simulink model "driver_model_curve"  (R2023b)
settings: Solver=FixedStepAuto  StartTime=0.0  StopTime=50  FixedStep=0.001  MaxStep=0.001  RelTol=1e-3
libraries: Solver_SF x1, slpidlib x1
settings Model: DataTypeOverride=Double  MinMaxOverflowLogging=ForceOff  Creator=황수빈  LastModifiedBy=황수빈

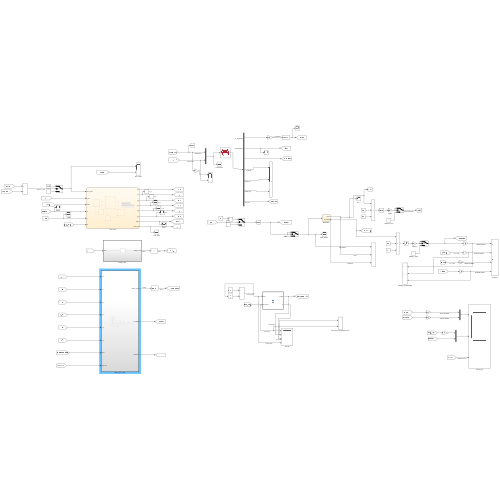
[thumbnail: Simulink's stored preview of the top-level diagram]
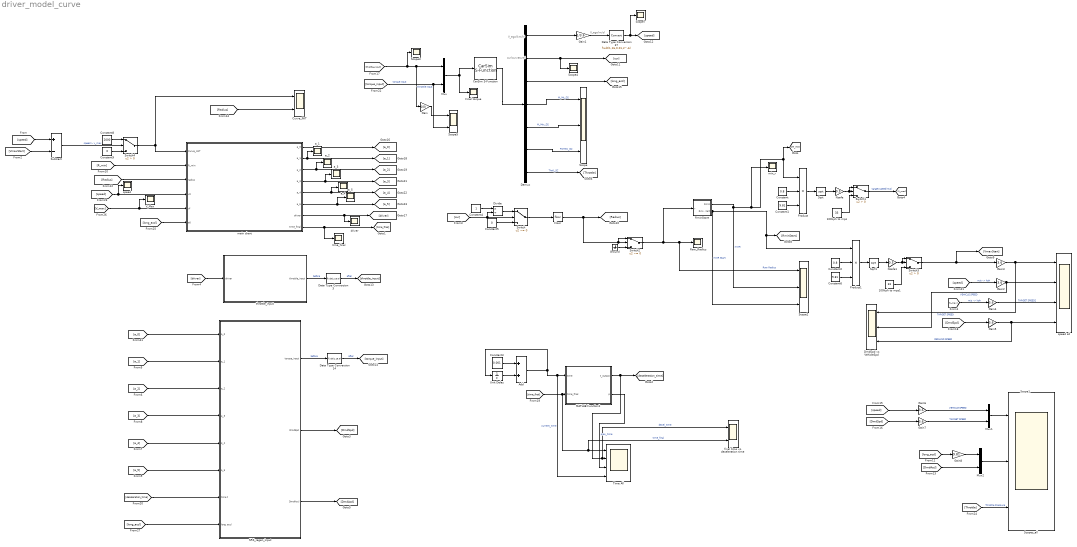
== system driver_model_curve ==
  note: V_ego(km/h)
  note: V_ego(m/s)
  note: cur(curvature)
  100kph to mps : Constant  Value=33
  100kph to mps1 : Constant  Value=33
  Add : Sum
  CarSim S-Function : Solver_SF/CarSim S-Function  Priority=1  SIMFILE=simfile.sim  Run_RTs=off  vs_state_ind=Run  StopMode_ind=Vehicle Model
  Constant : Constant  Value=0.8
  Constant1 : Constant  Value=9.81
  Constant2 : Constant  Value=0.8
  Constant3 : Constant  Value=0.001
  Constant4 : Constant
  Constant5 : Constant  Value=0
  Constant6 : Constant  Value=9.81
  Constant8 : Constant  Value=2000
  Constant9 : Constant  Value=0
  Curve_INIT : Scope  NumInputPorts=2
  Data Type Conversion14 : DataTypeConversion  OutDataTypeStr=fixdt(1,16,0)  RndMeth=Nearest  SaturateOnIntegerOverflow=off
  Data Type Conversion3 : DataTypeConversion  OutDataTypeStr=fixdt(1,16,0)  RndMeth=Nearest  SaturateOnIntegerOverflow=off
  Data Type Conversion37 : DataTypeConversion  OutDataTypeStr=fixdt(1,16,0.01,2^-6)  RndMeth=Simplest  SaturateOnIntegerOverflow=off
  Demux : Demux  Outputs=7
  Divide : Product  Inputs=*/
  DmdSpd vs VehicleSpd : Scope  NumInputPorts=3
  Final torque : Scope
  Floor : Rounding
  Gain : Gain  Gain=100
  Gain1 : Gain  Gain=1/3.6
  Gain{2..7} (6 alike) : Gain  Gain=3.6
  Gain8 : Gain  Gain=9.81
  Ground : Ground
  MATLAB Function1 : MATLAB Function  TreatAsAtomicUnit=on
  Mux : Mux  Inputs=2
  Mux1 : Mux  Inputs=2
  Mux2 : Mux  Inputs=2
  Nsafe : Gain  Gain=0.5
  Nsafe1 : Gain  Gain=0.5
  Product : Product  Inputs=3
  Product1 : Product  Inputs=3
  Raw_Radius : Scope
  RminStore : Stateflow chart  TreatAsAtomicUnit=on
  SRS_regen_input : Subsystem  TreatAsAtomicUnit=on
  Scope : Scope  NumInputPorts=3
  Scope{1,3..4,7} (4 alike) : Scope
  Scope2 : Scope  NumInputPorts=3
  Scope5 : Scope  NumInputPorts=2
  Scopes_all : Scope  NumInputPorts=3
  Sqrt : Sqrt
  Sqrt1 : Sqrt
  Subtract : Sum  Inputs=+-
  Switch : Switch  Criteria=u2 ~= 0  SaturateOnIntegerOverflow=off  InputSameDT=off
  Switch1 : Switch  Criteria=u2 > Threshold  SaturateOnIntegerOverflow=off  InputSameDT=off
  Switch2 : Switch  Criteria=u2 ~= 0  SaturateOnIntegerOverflow=off  InputSameDT=off
  Switch3 : Switch  Criteria=u2 > Threshold  SaturateOnIntegerOverflow=off  InputSameDT=off
  Switch4 : Switch  Criteria=u2 > Threshold  SaturateOnIntegerOverflow=off  InputSameDT=off
  Time All : Scope  NumInputPorts=4
  Unit Delay : UnitDelay  SampleTime=-1  HasFrameUpgradeWarning=on
  V_Max : Scope
  a_{1..5} (5 alike) : Scope
  driver : Scope
  final time vs. deceleration time : Scope  NumInputPorts=2
  main chart : Stateflow chart  TreatAsAtomicUnit=on
  min_r : Scope
  speed : Scope
  speed all : Scope  NumInputPorts=4
  throttle_input : Subsystem  TreatAsAtomicUnit=on  SystemSampleTime=0.01
  time_final : Scope
  wires:
  Switch/1 -> Floor/1
  [cur] -> Switch/2, Divide/2
  Constant5/1 -> Switch/3
  Constant4/1 -> Divide/1
  Divide/1 -> Switch/1
  Gain1/1 -> Data Type Conversion37/1
  Demux/1 -> Gain1/1
  Demux/2 -> Scope4/1, [cur]
  Data Type Conversion37/1 -> Scope7/1, [speed]
  CarSim S-Function/1 -> Demux/1
  [driver] -> throttle_input/1(driver)
  Data Type Conversion3/1 -> [throttle_input]  "after"
  throttle_input/1(throttle_input) -> Data Type Conversion3/1  "before"
  SRS_regen_input/1(torque_input) -> Data Type Conversion14/1  "before"
  [a_2] -> SRS_regen_input/3(a_2)
  Data Type Conversion14/1 -> [torque_input]  "after"
  [a_0] -> SRS_regen_input/1(a_0)
  [a_3] -> SRS_regen_input/4(a_3)
  [a_5] -> SRS_regen_input/6(a_5)
  Demux/3 -> [long_accl]
  [a_1] -> SRS_regen_input/2(a_1)
  [a_4] -> SRS_regen_input/5(a_4)
  Constant8/1 -> Switch4/1
  Constant9/1 -> Switch4/3
  Switch4/1 -> main chart/1(Curve_INIT), Curve_INIT/1
  [speed] -> main chart/4(v0), speed/1
  [V_max] -> V_Max/1, main chart/5(vf)
  main chart/3(a_2) -> a_2/1, [a_2]
  main chart/4(a_3) -> a_3/1, [a_3]
  main chart/5(a_4) -> a_4/1, [a_4]
  main chart/2(a_1) -> a_1/1, [a_1]
  main chart/6(a_5) -> a_5/1, [a_5]
  main chart/7(driver) -> driver/1, [driver]
  [V_max] -> Gain4/1  "m/s -> kph"
  [speed] -> Subtract/1
  [VmaxStart] -> Subtract/2
  Subtract/1 -> Switch4/2  "speed > v_max"
  [R_min] -> main chart/2(R_min)
  main chart/8(time_final) -> time_final/1, [time_final]
  Add/1 -> Unit Delay/1, Time All/4, MATLAB Function1/1(time)  "current_time"
  Gain2/1 -> DmdSpd vs VehicleSpd/2, speed all/2  "VEHICLE SPEED"
  [speed] -> Gain2/1  "m/s -> kph"
  [time_final] -> final time vs. deceleration time/2, Time All/1, MATLAB Function1/2(time_final)  "time_final"
  [Radius] -> main chart/3(radius)
  [torque_input] -> Mux/2, Scope5/2  "torque input"
  [throttle_input] -> Scope3/1, Gain/1, Mux/1  "throttle input"
  Mux/1 -> Final torque/1, CarSim S-Function/1
  Constant3/1 -> Add/1
  Unit Delay/1 -> Add/2
  MATLAB Function1/1(t_output) -> final time vs. deceleration time/1, Time All/2, [deceleration_time]  "decel_time"
  main chart/1(a_0) -> [a_0]
  Constant1/1 -> Product/3
  100kph to mps/1 -> Switch1/3
  Product/1 -> Sqrt/1
  Constant/1 -> Product/2
  Sqrt/1 -> Nsafe/1
  Nsafe/1 -> Switch1/1, Switch1/2
  Switch2/1 -> Scope2/1, Raw_Radius/1, RminStore/1(r)  "Raw Radius"
  Switch1/1 -> [V_max]  "target speed(m/s)"
  Floor/1 -> Switch2/1, Switch2/2, [Radius]
  Ground/1 -> Switch2/3
  MATLAB Function1/2(p) -> Time All/3  "prev_time"
  [deceleration_time] -> SRS_regen_input/7(time t)
  [long_accl] -> main chart/6(a0)
  [long_accl] -> SRS_regen_input/8(long. accl)
  [Radius] -> Curve_INIT/2
  Nsafe1/1 -> Switch3/1, Switch3/2
  100kph to mps1/1 -> Switch3/3
  Constant6/1 -> Product1/3
  Sqrt1/1 -> Nsafe1/1
  Constant2/1 -> Product1/2
  Product1/1 -> Sqrt1/1
  RminStore/1(Rmin) -> min_r/1, Product/1, [R_min], Scope2/2  "minR"
  Switch3/1 -> [VmaxStart], Gain3/1
  Gain3/1 -> DmdSpd vs VehicleSpd/1, speed all/1  "TARGET SPEED"
  SRS_regen_input/2(DmdSpd) -> [DmdSpd]
  [DmdSpd] -> Gain5/1
  Gain5/1 -> DmdSpd vs VehicleSpd/3, speed all/4  "DEMAND SPEED"
  Gain4/1 -> speed all/3  "TARGET SPEED2"
  RminStore/2(RminStart) -> Scope2/3, [RminStart], Product1/1  "minR Start"
  Demux/4 -> Scope/1  "M_Mt_D2"
  Demux/5 -> Scope/2  "M_Mtr_D2"
  Demux/6 -> Scope/3  "PwMtC_D2"
  Demux/7 -> [Throttle]  "Thrtl_SC"
  Gain/1 -> Scope5/1
  SRS_regen_input/3(DmdAccl) -> [DmdAccl]
  [long_accl] -> Gain8/1
  [speed] -> Gain6/1
  [DmdSpd] -> Gain7/1
  Gain7/1 -> Mux1/2  "TARGET SPEED"
  Gain6/1 -> Mux1/1  "VEHICLE SPEED"
  [DmdAccl] -> Mux2/2
  Gain8/1 -> Mux2/1
  Mux1/1 -> Scopes_all/1
  Mux2/1 -> Scopes_all/2
  [Throttle] -> Scopes_all/3  "Throttle Pressure"

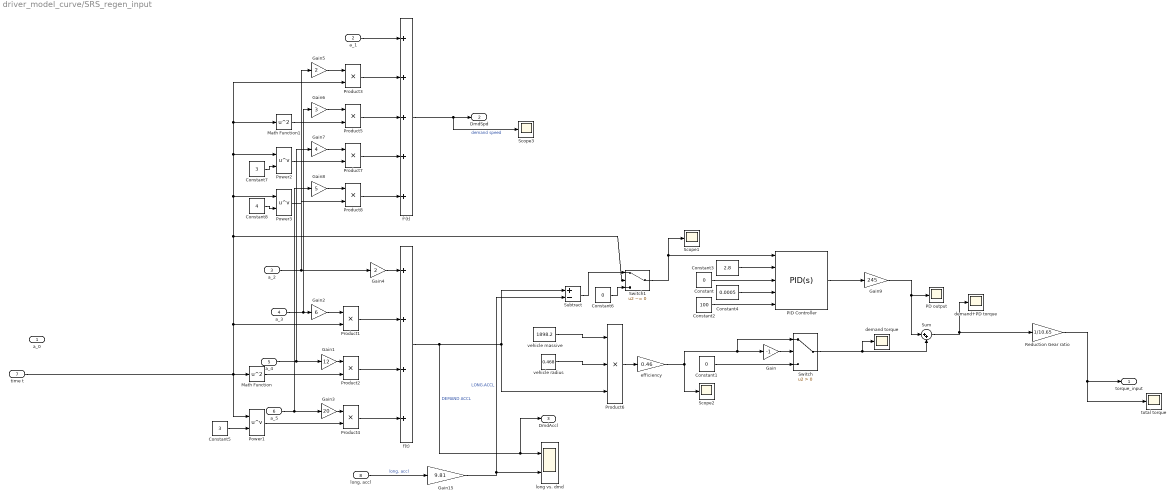
== system driver_model_curve/SRS_regen_input ==
  a_0 : Inport
  a_1 : Inport  Port=2
  a_2 : Inport  Port=3
  a_3 : Inport  Port=4
  a_4 : Inport  Port=5
  a_5 : Inport  Port=6
  time t : Inport  Port=7
  long. accl : Inport  Port=8
  Constant : Constant  Value=0
  Constant1 : Constant  Value=0
  Constant2 : Constant  Value=100
  Constant3 : Constant  Value=2.8
  Constant4 : Constant  Value=0.0005
  Constant5 : Constant  Value=3
  Constant6 : Constant  Value=0
  Constant7 : Constant  Value=3
  Constant8 : Constant  Value=4
  Gain : Gain  Gain=-1
  Gain1 : Gain  Gain=12
  Gain15 : Gain  Gain=9.81
  Gain2 : Gain  Gain=6
  Gain3 : Gain  Gain=20
  Gain4 : Gain  Gain=2
  Gain5 : Gain  Gain=2
  Gain6 : Gain  Gain=3
  Gain7 : Gain  Gain=4
  Gain8 : Gain  Gain=5
  Gain9 : Gain  Gain=245
  Math Function : Math  Operator=square
  Math Function1 : Math  Operator=square
  PD output : Scope
  PID Controller : slpidlib/PID Controller  Controller=PID  Form=Parallel  TimeDomain=Continuous-time  UseExternalTs=off  SampleTime=-1  IntegratorMethod=Forward Euler  FilterMethod=Forward Euler  ControllerParametersSource=external  P=1  I=1  UseKiTs=off  D=0  N=100  UseFilter=on  TunerSelectOption=Transfer Function Based (PID Tuner App)  InitialConditionSource=internal  InitialConditionForIntegrator=0  InitialConditionForFilter=0  DifferentiatorICPrevScaledInput=0  ExternalReset=none  TrackingMode=off  Kt=1  LimitOutput=off  SatLimitsSource=internal  UpperSaturationLimit=inf  LowerSaturationLimit=-inf  LinearizeAsGain=on  AntiWindupMode=none  Kb=1  LimitIntegrator=off  UpperIntegratorSaturationLimit=inf  LowerIntegratorSaturationLimit=-inf  POutMin=[]  POutMax=[]  IOutMin=[]  IOutMax=[]  DOutMin=[]  DOutMax=[]  NOutMin=[]  NOutMax=[]  SumOutMin=[]  SumOutMax=[]  SaturationOutMin=[]  SaturationOutMax=[]  PParamMin=[]  PParamMax=[]  IParamMin=[]  IParamMax=[]  DParamMin=[]  DParamMax=[]  NParamMin=[]  NParamMax=[]  KbParamMin=[]  KbParamMax=[]  KtParamMin=[]  KtParamMax=[]  KbOutMin=[]  KbOutMax=[]  KtOutMin=[]  KtOutMax=[]  IntegratorOutMin=[]  IntegratorOutMax=[]  FilterOutMin=[]  FilterOutMax=[]  SumI1OutMin=[]  SumI1OutMax=[]  SumI2OutMin=[]  SumI2OutMax=[]  SumI3OutMin=[]  SumI3OutMax=[]  SumI4OutMin=[]  SumI4OutMax=[]  SumDOutMin=[]  SumDOutMax=[]  DifferentiatorOutMin=[]  DifferentiatorOutMax=[]  FilterDiffOutCoefMin=[]  FilterDiffOutCoefMax=[]  ReciprocalOutMin=[]  ReciprocalOutMax=[]  SumDenOutMin=[]  SumDenOutMax=[]  SumNumOutMin=[]  SumNumOutMax=[]  DivideOutMin=[]  DivideOutMax=[]  UdiffTsProdOutMin=[]  UdiffTsProdOutMax=[]  NTsProdOutMin=[]  NTsProdOutMax=[]  UintegralTsProdOutMin=[]  UintegralTsProdOutMax=[]  UngainTsProdOutMin=[]  UngainTsProdOutMax=[]  ClampingZeroOutDataTypeStr=Inherit: Inherit via back propagation  ClampingZeroOutMin=[]  ClampingZeroOutMax=[]  FilterDenConstantOutDataTypeStr=Inherit: Inherit via back propagation  FilterDenConstantOutMin=[]  FilterDenConstantOutMax=[]  PCopyOutDataTypeStr=Inherit: Inherit via back propagation  PCopyOutMin=[]  PCopyOutMax=[]  NCopyOutDataTypeStr=Inherit: Inherit via back propagation  NCopyOutMin=[]  NCopyOutMax=[]  IntegratorContinuousStateAttributes=''  IntegratorStateMustResolveToSignalObject=off  IntegratorRTWStateStorageClass=Auto  FilterContinuousStateAttributes=''  FilterStateMustResolveToSignalObject=off  FilterRTWStateStorageClass=Auto  ParallelPVariant=ExternalParameters  IdealPVariant=Disabled  IVariant=ExternalParameters  DVariant=ExternalParameters  IntegratorVariant=Continuous  SatVariant=Disabled  AWVariant=Passthrough  PCopyVariant=Disabled  TRVariant=Disabled  FdbkBlocksVariant=Forward  IdealPFdbkVariant=Disabled  SatFdbkVariant=Disabled  DerivativeFilterVariant=ContFilter  NVariant=ExternalParameters  NCopyVariant=Disabled  FilterICVariant=InternalICsFilter  IntegratorICVariant=InternalICs  ExternalResetVariant=Disabled  TRSumVariant=Passthrough  SumFdbkVariant=Disabled  SumVariant=Sum_PID  TsampFilterVariant=InternalTs  TsampNgainVariant=Passthrough  TsampIntegralVariant=Disabled_SignalSpec  ExternalSaturationOutDataTypeStr=Inherit: Same as second input
  Power1 : Math  Operator=pow
  Power2 : Math  Operator=pow
  Power3 : Math  Operator=pow
  Product{1..5,7..8} (7 alike) : Product
  Product6 : Product  Inputs=3
  Reduction Gear ratio : Gain  Gain=1/10.65
  Scope1 : Scope
  Scope2 : Scope
  Scope3 : Scope
  Subtract : Sum  Inputs=+-
  Sum : Sum  Inputs=|++
  Switch : Switch  Criteria=u2 > Threshold  SaturateOnIntegerOverflow=off  InputSameDT=off
  Switch1 : Switch  Criteria=u2 ~= 0  SaturateOnIntegerOverflow=off  InputSameDT=off
  demand torque : Scope
  demand+PD torque : Scope
  efficiency : Gain  Gain=0.46
  f'(t) : Sum  Inputs=5
  f(t) : Sum  Inputs=4
  long vs. dmd : Scope  NumInputPorts=2
  total torque : Scope
  vehicle massive : Constant  Value=1898.2
  vehicle radius : Constant  Value=0.468
  torque_input : Outport
  DmdSpd : Outport  Port=2
  DmdAccl : Outport  Port=3
  wires:
  time t/1 -> Power3/1, Power2/1, Math Function1/1, Product3/2, Switch1/2, Product1/2, Power1/1, Math Function/1
  Constant5/1 -> Power1/2
  Product2/1 -> f(t)/3
  Product4/1 -> f(t)/4
  Power1/1 -> Product4/2
  Math Function/1 -> Product2/2
  Product6/1 -> efficiency/1
  efficiency/1 -> Scope2/1, Switch/1, Gain/1
  Constant1/1 -> Switch/3
  Gain/1 -> Switch/2
  f(t)/1 -> Product6/3, Subtract/1, DmdAccl/1, long vs. dmd/1  "DEMAND ACCL"
  a_2/1 -> Gain4/1, Gain5/1
  a_4/1 -> Gain1/1, Gain7/1
  Gain1/1 -> Product2/1
  a_5/1 -> Gain8/1, Gain3/1
  Gain3/1 -> Product4/1
  Gain4/1 -> f(t)/1
  a_3/1 -> Gain6/1, Gain2/1
  Gain2/1 -> Product1/1
  Product1/1 -> f(t)/2
  long. accl/1 -> Gain15/1  "long. accl"
  Subtract/1 -> Switch1/1
  Switch1/1 -> PID Controller/1, Scope1/1
  Constant6/1 -> Switch1/3
  Constant2/1 -> PID Controller/5
  Constant4/1 -> PID Controller/4
  Constant/1 -> PID Controller/3
  Constant3/1 -> PID Controller/2
  PID Controller/1 -> Gain9/1
  a_1/1 -> f'(t)/1
  Product3/1 -> f'(t)/2
  Product5/1 -> f'(t)/3
  Product7/1 -> f'(t)/4
  Product8/1 -> f'(t)/5
  Gain5/1 -> Product3/1
  Gain6/1 -> Product5/1
  Gain7/1 -> Product7/1
  Gain8/1 -> Product8/1
  f'(t)/1 -> Scope3/1, DmdSpd/1  "demand speed"
  Math Function1/1 -> Product5/2
  Power2/1 -> Product7/2
  Power3/1 -> Product8/2
  Constant7/1 -> Power2/2
  Constant8/1 -> Power3/2
  Switch/1 -> Sum/2, demand torque/1
  Gain15/1 -> Subtract/2, long vs. dmd/2  "LONG.ACCL"
  vehicle radius/1 -> Product6/2
  vehicle massive/1 -> Product6/1
  Sum/1 -> Reduction Gear ratio/1, demand+PD torque/1
  Gain9/1 -> PD output/1, Sum/1
  Reduction Gear ratio/1 -> total torque/1, torque_input/1

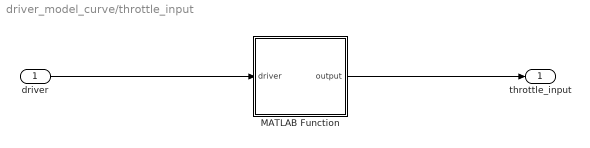
== system driver_model_curve/throttle_input ==
  driver : Inport
  MATLAB Function : MATLAB Function  TreatAsAtomicUnit=on
  throttle_input : Outport
  wires:
  driver/1 -> MATLAB Function/1(driver)
  MATLAB Function/1(output) -> throttle_input/1

== matlab function driver_model_curve/MATLAB Function1 ==
  data: time input; t_output output; time_final input; p output
function [t_output, p] = fcn(time, time_final)
    persistent prev_time;  % 이전 시간 저장용 변수
    if isempty(prev_time)
        prev_time = time;  % 초기화, 첫 호출 시 현재 시간으로 설정
    end

    % time이 time_final에 도달하면 prev_time을 초기화
    if (time - prev_time) < time_final 
        t_output = (time - prev_time);  % time_final에 도달하기 전까지의 값
        p = prev_time;

    
    elseif (time - prev_time) == time_final 
        t_output = 0;  % time_final에 도달하기 전까지의 값
        p = prev_time;

    else
        prev_time = time;  % 새로운 loop 시작 (time_final 도달 후 초기화)
        t_output = 0;  % time_final 도달 후 초기화된 slow_time
        p = prev_time;

    end

end

== matlab function driver_model_curve/throttle_input/MATLAB Function ==
  data: driver input; output output
function output = driver_function(driver)
    switch driver
        case 0
            output = 0;
        case 1
            output = 0.4;
        case 2
            output = 0.04;
        otherwise
            output = 0.4;
    end
end

== stateflow chart driver_model_curve/RminStore ==
  state RminStopStoring
    Rmin = minimum;
    RminStart = 0;
  state RminStoring
    if r>2500 && r<3000
    minimum = r-2500;
    end
    Rmin = minimum;
    RminStart = minimum;
  state INITIAL
    minimum = 0;
    Rmin=0;
    RminStart=0;
  (default) -> INITIAL
  INITIAL -> RminStoring : [r > 2500 && r < 3000]
  RminStoring -> RminStopStoring : [minimum == r]
  (junction 14) -> INITIAL
  RminStopStoring -> (junction 14) : [minimum < r]
  data: r input; Rmin output; minimum local; RminStart output

== stateflow chart driver_model_curve/main chart ==
  state CurveRoadState
    during:
    driver = 0;
    if (radius-2500 == R_min )
    if v0 ~= 0
    if (flag_v == 0)
    vv = v0;
    flag_v = 1;
    end
    end
    [distance, time_final] = var_cal(R_min, vv, vf);
    if distance ~= 0
    dd = distance;
    end
    if time_final ~= 0
    tt = time_final;
    end
    if v0 ~= 0
    if (flag_a == 0)
    aa = a0;
    flag_a = 1;
    end
    end
    [a_0, a_1, a_2, a_3, a_4, a_5] = calculate(vv,aa,vf,dd,tt);
    else
    flag_v = 0;
    flag_a = 0;
    end
  state InitialState
    driver = 0;
    aa = 0;
    vv = 0;
    dd = 0;
    tt = 0;
    flag_v = 0;
    flag_a = 0;
  state KeepSpdState
    driver = 2;
    distance = 0;
    time_final = 0;
    a_0=0;
    a_1=0;
    a_2=0;
    a_3=0;
    a_4=0;
    a_5=0;
    vv=0;
    aa=0;
  state PowerAccelState
    driver = 3;
  state NormAccelState
    driver = 1;
  (default) -> InitialState
  CurveRoadState -> (junction 83) : [Curve_INIT==0]
  InitialState -> CurveRoadState [order 1] : [Curve_INIT ~= 0 ]
  (junction 83) -> KeepSpdState
  (junction 87) -> CurveRoadState
  PowerAccelState -> (junction 87) : [Curve_INIT ~= 0]
  InitialState -> (junction 46) [order 2] : [Curve_INIT==0]
  NormAccelState -> CurveRoadState : [Curve_INIT ~= 0]
  (junction 46) -> PowerAccelState
  KeepSpdState -> (junction 85) : [radius > R_min]
  (junction 85) -> NormAccelState
  data: R_min function_input; distance function_output; time_final function_output; v0 function_input; vf function_input; v0 function_input; a0 function_input; vf function_input; a_0 function_output; a_1 function_output; a_2 function_output; a_3 function_output; a_4 function_output; a_5 function_output; distance function_input; time_final function_input; Curve_INIT input; R_min input; radius input; v0 input; vf input; a_0 output; a_1 output; a_2 output; a_3 output; a_4 output; a_5 output; driver output; time_final output; tt local; aa local; dd local; distance local; a0 input; flag_v local; flag_a local; vv local
  function [distance, time_final] = var_cal(R_min, v0, vf):
    | function [distance, time_final] = var_cal(R_min, v0, vf)
    |     % radius: 입력 값
    |     % v0: 초기 속도
    |     % vf: 최종 속도
    |     % distance: 조건에 따른 결과 값
    |     % tf: 계산된 시간 (distance / ((v0 + vf) / 2))
    | 
    |     %a_target = (a0 + 0) / 2;
    | 
    |     % 조건에 따라 distance 설정
    |     if R_min == 56
    |         distance = 266.5;
    |     elseif R_min == 108
    |         distance = 84;
    |     elseif R_min == 220
    |         distance = 138.5;
    |             % 기본 값 설정
    |     else
    |             distance = NaN;  % 유효한 값이 없을 때 NaN 반환
    |     end
    |     
    |     % tf 계산 (distance가 NaN이 아니면 계산)
    |     if ~isnan(distance)
    |         %a_final = a_target + a_slope;
    |         %time_final = (vf - v0) / a_final;
    |         time_final = distance / ((v0 + vf) / 2);  % 평균 속도를 사용하여 시간 계산
    |     else
    |         time_final = NaN;  % distance가 유효하지 않으면 tf도 NaN으로 설정
    |     end
    | end
  function [a_0, a_1, a_2, a_3, a_4, a_5] =  calculate(v0, a0, vf, distance, time_final):
    | function [a_0, a_1, a_2, a_3, a_4, a_5] =  calculate(v0, a0, vf, distance, time_final)
    | 
    | %% 5차 profiling %%
    | xf = distance;
    | tf = time_final;
    | af = 0; %임의로 지정
    | 
    | A = [1, 0, 0, 0, 0, 0;
    |     0, 1, 0, 0, 0, 0;
    |     0, 0, 2, 0, 0, 0;
    |     1, tf, tf^2, tf^3, tf^4, tf^5;
    |     0, 1, 2*tf, 3*tf^2, 4*tf^3, 5*tf^4;
    |     0, 0, 2, 6*tf, 12*tf^2, 20*tf^3;];
    | 
    | B = [0; v0; a0; xf; vf; af;];
    | 
    | % 연립 방정식 풀기 (A \ B 사용)
    | coeffs = A \ B;
    | 
    | % 계수 추출
    | a_0 = coeffs(1);
    | a_1 = coeffs(2);
    | a_2 = coeffs(3);
    | a_3 = coeffs(4);
    | a_4 = coeffs(5);
    | a_5 = coeffs(6);
